simulink model "ans2_65070121_155_168"  (R2024b)
settings: Solver=ode8  StartTime=0  StopTime=19  FixedStep=0.001  RelTol=1e-3
settings Model: Creator=picha  LastModifiedBy=picha

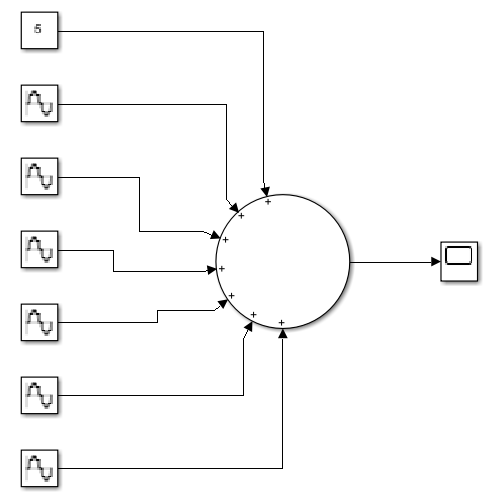
[thumbnail: Simulink's stored preview of the top-level diagram]
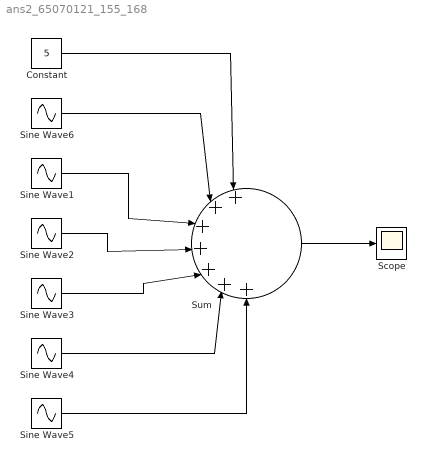
== system ans2_65070121_155_168 ==
  Constant : Constant  Value=5
  Scope : Scope
  Sine Wave1 : Sin  Amplitude=4/(3*pi)  Frequency=3  Phase=2*pi  SampleTime=0.001
  Sine Wave2 : Sin  Amplitude=4/(5*pi)  Frequency=5  Phase=2*pi  SampleTime=0.001
  Sine Wave3 : Sin  Amplitude=4/(7*pi)  Frequency=7  Phase=2*pi  SampleTime=0.001
  Sine Wave4 : Sin  Amplitude=4/(9*pi)  Frequency=9  Phase=2*pi  SampleTime=0.001
  Sine Wave5 : Sin  Amplitude=4/(11*pi)  Frequency=11  Phase=2*pi  SampleTime=0.001
  Sine Wave6 : Sin  Amplitude=4/pi  Phase=2*pi  SampleTime=0.001
  Sum : Sum  Inputs=|+|+|+|+|+|+|+
  wires:
  Constant/1 -> Sum/1
  Sine Wave6/1 -> Sum/2
  Sine Wave1/1 -> Sum/3
  Sine Wave2/1 -> Sum/4
  Sine Wave3/1 -> Sum/5
  Sine Wave4/1 -> Sum/6
  Sine Wave5/1 -> Sum/7
  Sum/1 -> Scope/1
